simulink model "Steer_example"  (R2016b)
settings: Solver=VariableStepAuto  StartTime=0.0  StopTime=inf  RelTol=1e-3
undefined symbols (not defined in the file): serial
libraries: instrumentlib x2
settings Model: Creator=AK-47  LastModifiedBy=AK-47

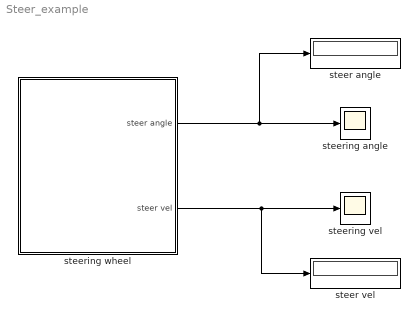
== system Steer_example ==
  steer angle : Display
  steer vel : Display
  steering angle : Scope
  steering vel : Scope
  steering wheel : Subsystem
      mask Display: image('C:\Users\AK-47\Desktop\New folder (2)\612sNJ+2VVL._AC_SX355_.jpg');
  wires:
  steering wheel/1(steer angle) -> steering angle/1, steer angle/1
  steering wheel/2(steer vel) -> steer vel/1, steering vel/1

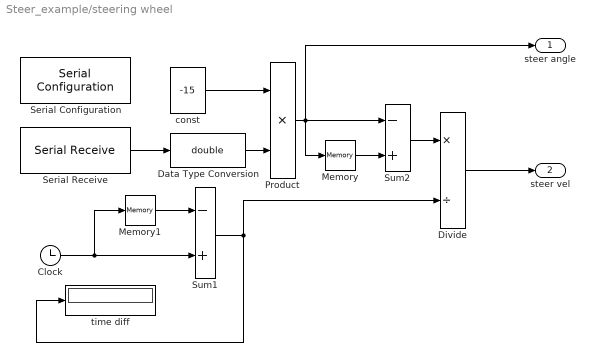
== system Steer_example/steering wheel ==
  Clock : Clock
  Data Type Conversion : DataTypeConversion  OutDataTypeStr=double
  Divide : Product  Inputs=*/
  Memory : Memory
  Memory1 : Memory
  Product : Product
  Serial Configuration : instrumentlib/Serial Configuration  Priority=-200000  ComPortMenu=COM3  ComPort=COM3  ObjConstructor=serial('COM3');  BaudRate=9600  DataBits=8  Parity=none  StopBits=1  FlowControl=none  Timeout=10  ByteOrder=LittleEndian
  Serial Receive : instrumentlib/Serial Receive  ComPortMenu=<Please select a port...>  ComPort=COM3  ObjConstructor=serial('COM3');  Terminator=<none>  DataSize=[1 1]  DataType=int8  EnableBlockingMode=on  ActionDataUnavailable=Output last received value  CustomValue=0  SampleTime=0.1
  Sum1 : Sum  Inputs=-+
  Sum2 : Sum  Inputs=-+
  "const " : Constant  Value=-15
  time diff : Display
  steer angle : Outport
  steer vel : Outport  Port=2
  wires:
  Product/1 -> Memory/1, Sum2/1, steer angle/1
  "const "/1 -> Product/1
  Sum2/1 -> Divide/1
  Serial Receive/1 -> Data Type Conversion/1
  Memory/1 -> Sum2/2
  Data Type Conversion/1 -> Product/2
  Clock/1 -> Memory1/1, Sum1/2
  Memory1/1 -> Sum1/1
  Sum1/1 -> time diff/1, Divide/2
  Divide/1 -> steer vel/1
